simulink model "tractionControlSystem"  (R2013a)
settings: Solver=ode45  StartTime=0.0  StopTime=10.0  MinStep=0.001  RelTol=1e-6
undefined symbols (not defined in the file or in its folder): driverDesired, XXXXXXXXXXXXXX
libraries: simulink x1
settings Model: Creator=YW Liao  LastModifiedBy=YW Liao

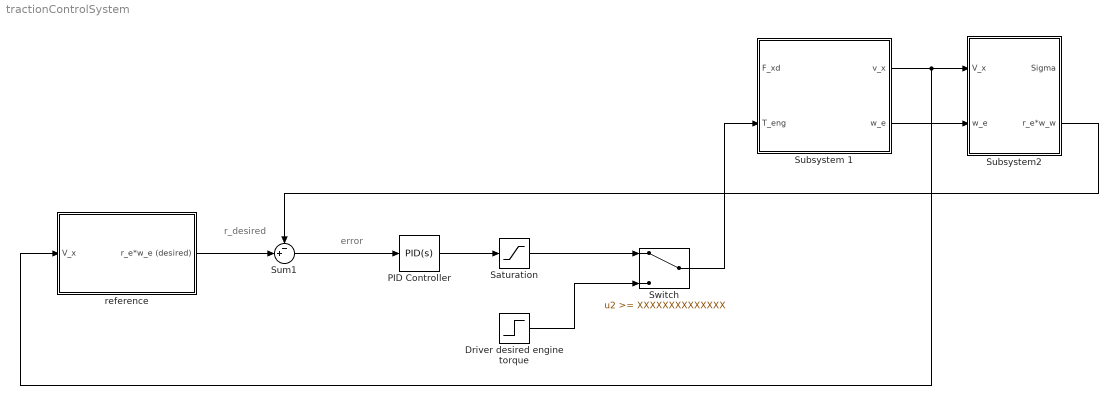
== system tractionControlSystem ==
  note: error
  note: r_desired
  Driver desired engine torque : Step  Time=0  After=driverDesired  SampleTime=0
  "PID Controller " : simulink/Continuous/PID Controller  Controller=PID  TimeDomain=Continuous-time  SampleTime=1  IntegratorMethod=Forward Euler  FilterMethod=Forward Euler  Form=Parallel  P=1  I=1  D=0  N=100  InitialConditionSource=internal  InitialConditionForIntegrator=0  InitialConditionForFilter=0  ExternalReset=none  LimitOutput=off  UpperSaturationLimit=inf  LowerSaturationLimit=-inf  LinearizeAsGain=on  AntiWindupMode=none  Kb=1  TrackingMode=off  Kt=1  PParamMin=[]  PParamMax=[]  IParamMin=[]  IParamMax=[]  DParamMin=[]  DParamMax=[]  NParamMin=[]  NParamMax=[]  KbParamMin=[]  KbParamMax=[]  KtParamMin=[]  KtParamMax=[]  POutMin=[]  POutMax=[]  IOutMin=[]  IOutMax=[]  DOutMin=[]  DOutMax=[]  NOutMin=[]  NOutMax=[]  KbOutMin=[]  KbOutMax=[]  KtOutMin=[]  KtOutMax=[]  IntegratorOutMin=[]  IntegratorOutMax=[]  FilterOutMin=[]  FilterOutMax=[]  SumOutMin=[]  SumOutMax=[]  SumI1OutMin=[]  SumI1OutMax=[]  SumI2OutMin=[]  SumI2OutMax=[]  SumI3OutMin=[]  SumI3OutMax=[]  SumDOutMin=[]  SumDOutMax=[]  SaturationOutMin=[]  SaturationOutMax=[]  IntegratorContinuousStateAttributes=''  IntegratorStateMustResolveToSignalObject=off  IntegratorRTWStateStorageClass=Auto  FilterContinuousStateAttributes=''  FilterStateMustResolveToSignalObject=off  FilterRTWStateStorageClass=Auto
  Saturation : Saturate  UpperLimit=180  LowerLimit=-30
  Subsystem 1 : Subsystem
  Subsystem2 : Subsystem
  Sum1 : Sum  Inputs=-+|
  Switch : Switch  Threshold=XXXXXXXXXXXXXX  ZeroCross=off
  reference : Subsystem
  wires:
  Sum1/1 -> "PID Controller "/1
  Subsystem 1/1(v_x) -> Subsystem2/1(V_x), reference/1(V_x)
  "PID Controller "/1 -> Saturation/1
  Subsystem2/2(r_e*w_w) -> Sum1/1
  Subsystem 1/2(w_e) -> Subsystem2/2(w_e)
  Driver desired engine torque/1 -> Switch/3
  Saturation/1 -> Switch/1
  reference/1(r_e*w_e (desired)) -> Sum1/2
  Switch/1 -> Subsystem 1/2(T_eng)

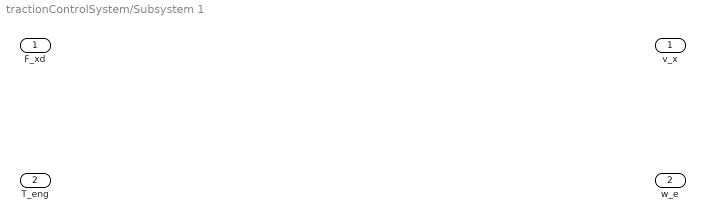
== system tractionControlSystem/Subsystem 1 ==
  F_xd : Inport
  T_eng : Inport  Port=2
  v_x : Outport
  w_e : Outport  Port=2

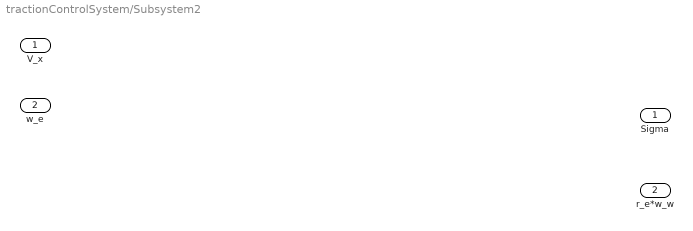
== system tractionControlSystem/Subsystem2 ==
  V_x : Inport
  w_e : Inport  Port=2
  Sigma : Outport
  r_e*w_w : Outport  Port=2

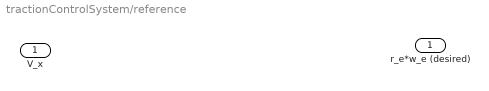
== system tractionControlSystem/reference ==
  V_x : Inport
  r_e*w_e (desired) : Outport
